simulink model "adder_code_gen"  (R2017b)
settings: Solver=FixedStepDiscrete  StartTime=0.0  StopTime=200  FixedStep=1  RelTol=1e-3
libraries: simulink x1
settings Model: Creator=roman  LastModifiedBy=roman

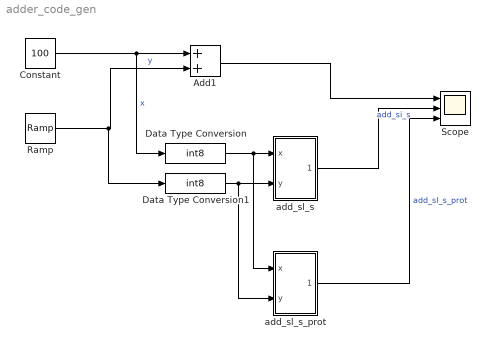
== system adder_code_gen ==
  Add1 : Sum  AccumDataTypeStr=double  OutDataTypeStr=Inherit: Same as accumulator
  Constant : Constant  Value=100
  Data Type Conversion : DataTypeConversion  OutDataTypeStr=int8
  Data Type Conversion1 : DataTypeConversion  OutDataTypeStr=int8
  Ramp : simulink/Sources/Ramp  slope=1  start=0  X0=0
  Scope : Scope  NumInputPorts=3
  add_sl_s : Subsystem
  add_sl_s_prot : Subsystem
  wires:
  Constant/1 -> Data Type Conversion/1, Add1/1  "x"
  Ramp/1 -> Data Type Conversion1/1, Add1/2  "y"
  Add1/1 -> Scope/1
  Data Type Conversion/1 -> add_sl_s_prot/1(x), add_sl_s/1(x)
  Data Type Conversion1/1 -> add_sl_s_prot/2(y), add_sl_s/2(y)
  add_sl_s/1(sum) -> Scope/2  "add_si_s"
  add_sl_s_prot/1(sum) -> Scope/3  "add_sl_s_prot"

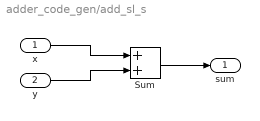
== system adder_code_gen/add_sl_s ==
  x : Inport
  y : Inport  Port=2
  Sum : Sum  AccumDataTypeStr=int8  OutDataTypeStr=Inherit: Same as accumulator
  sum : Outport
  wires:
  y/1 -> Sum/2
  Sum/1 -> sum/1
  x/1 -> Sum/1

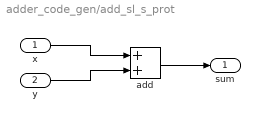
== system adder_code_gen/add_sl_s_prot ==
  x : Inport
  y : Inport  Port=2
  add : Sum  AccumDataTypeStr=int8  OutDataTypeStr=Inherit: Same as accumulator  SaturateOnIntegerOverflow=on
  sum : Outport
  wires:
  y/1 -> add/2
  add/1 -> sum/1
  x/1 -> add/1
